simulink library "MuteBtc"  (R2022b)
settings: Solver=VariableStepAuto  StartTime=0.0  StopTime=10.0  RelTol=1e-3
libraries: HandyTextFile x1, MuteControlBtc x1, MuteRamperBtc x1
settings Model: Creator=st51187  LastModifiedBy=kl13806
settings SolverCC: AlgebraicLoopSolver=TrustRegion
settings DebuggingCC: UnconnectedInputMsg=warning  UnconnectedOutputMsg=warning  UnconnectedLineMsg=warning  SFMachineParentedDataDiag=warning
settings ModelReferenceCC: EnableRefExpFcnMdlSchedulingChecks=on
settings RTWCC: DLArmComputeVersion=19.05

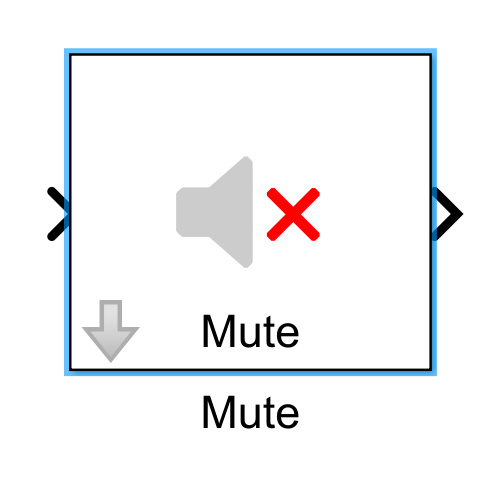
[thumbnail: Simulink's stored preview of the top-level diagram]
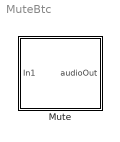
== system MuteBtc ==
  Mute : Subsystem  mask(Blocklib Mute){Config=[], FeatureName=Mute}
      mask prompts: Config "MuteConfig"; FeatureName "Mask feature name:"
      mask help: This block offers a simple mute feature using rgainy block. Set initial mute state for system cold start and a feature path name as desired. There are no tunable components, but runtime control is included.
      mask init:
      | blkh=gcbh;
      | Config=BTConfig.Assert(blkh,Config);
      | BTConfig.InitSetFeatureIfPresent(blkh,'FeatureName');
      | Config.Validate();
      mask Help:
      | This block offers a simple mute feature using rgainy block. The initial mute status of the block can be set through the mask.
      | 
      | RTC CONTROL:
      | Run time control is available to dynamically mute the audio. The mute status can be provided ('1' to mute audio), along with a ramp time and rate (rate gets precedence).
      | RTC_SIM_OBJ.AddREQ( 'MuteSet', 0.6, [0005,  <mute_status>, <ramp_db_per_second>, <ramp_time>]);
      | E.g., RTC_SIM_OBJ.AddREQ( 'MuteSet', 0.7, [0002, 1, 0, 50]);
      mask Callback Config: BTConfig.CallbackHideIfPresent(gcbh,{'FeatureName'});
      mask TypeOptions FeatureName: MuteControl/FeatureName | MuteRamper/FeatureName
      mask Display:
      | [path,w,h] = IconMuteMask();
      | 
      | % work in pixels since the icon does not scale
      | pos = get(gcbh,'position');
      | bw = pos(3) - pos(1);
      | bh = pos(4) - pos(2);
      | 
      | % Draw centered icon
      | xAdj = bw/2 - w/2;
      | yAdj = bh/2 - h/2;
      | for i=1:length(path)
      |     if (path(i).rgb(1) >= 0)
      |         patch(path(i).x+xAdj, path(i).y+yAdj, path(i).rgb);
      |     end
      |     if (path(i).stroke(1) >= 0)
      |         plot(path(i).x+xAdj, path(i).y+yAdj);
      |     end
      | end
      | 
      | % Display some text
      | text(bw/2, 2,FeatureName, ...
      |     'horizontalAlignment','center', ...
      |     'VerticalAlignment','bottom');

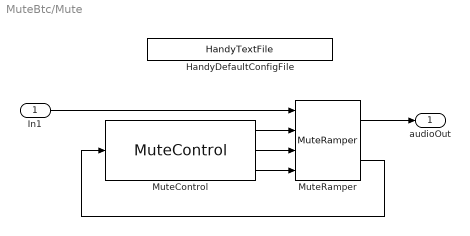
== system MuteBtc/Mute ==
  In1 : Inport
  HandyDefaultConfigFile : HandyTextFile/HandyTextFile  TemplateSource=Config  FileSuffix=Init  OpenDialogOnLoad=off  UseThisBlockName=off  AddGrandParentNamePrefix=off  TheDefaultText=|  ShowInLibBrowser=on
      | % $(FILENAME) Setup model parameters for each "Init" callback (e.g. update diagram)
      | sample_rate_in_hertz = 44100;
      | frame_size = 32;
      | sysin_channel_count = 2;
      settings: SourceProductName=Bose Talaria
  MuteControl : MuteControlBtc/MuteControl  Config=Config  FeatureName=Mute
      settings: SourceProductName=Bose Blocklib
  MuteRamper : MuteRamperBtc/MuteRamper  Config=Config  FeatureName=Mute
      settings: SourceProductName=Bose Blocklib
  audioOut : Outport
  wires:
  MuteControl/1 -> MuteRamper/2
  MuteControl/2 -> MuteRamper/3
  MuteControl/3 -> MuteRamper/4
  MuteRamper/2 -> MuteControl/1
  MuteRamper/1 -> audioOut/1
  In1/1 -> MuteRamper/1
